simulink model "IEEEG1_unitStepResponse"  (R2022a)
settings: Solver=VariableStepAuto  StartTime=0.0  StopTime=t_sim  RelTol=1e-3
undefined symbols (not defined in the file or in its folder): K, K1, K3, K5, K7, T1, T2, T3, T4, T5, T6, T7
settings Model: Creator=jongoh  LastModifiedBy=jongoh

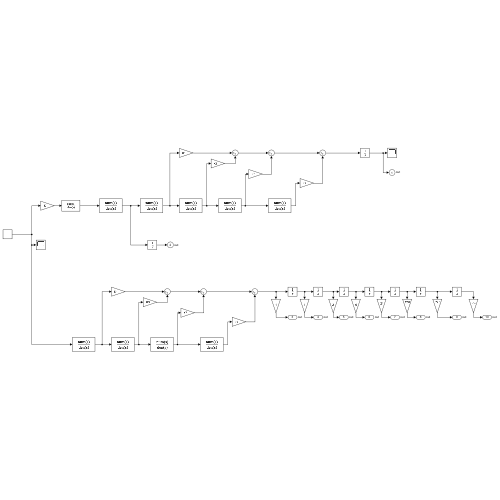
[thumbnail: Simulink's stored preview of the top-level diagram]
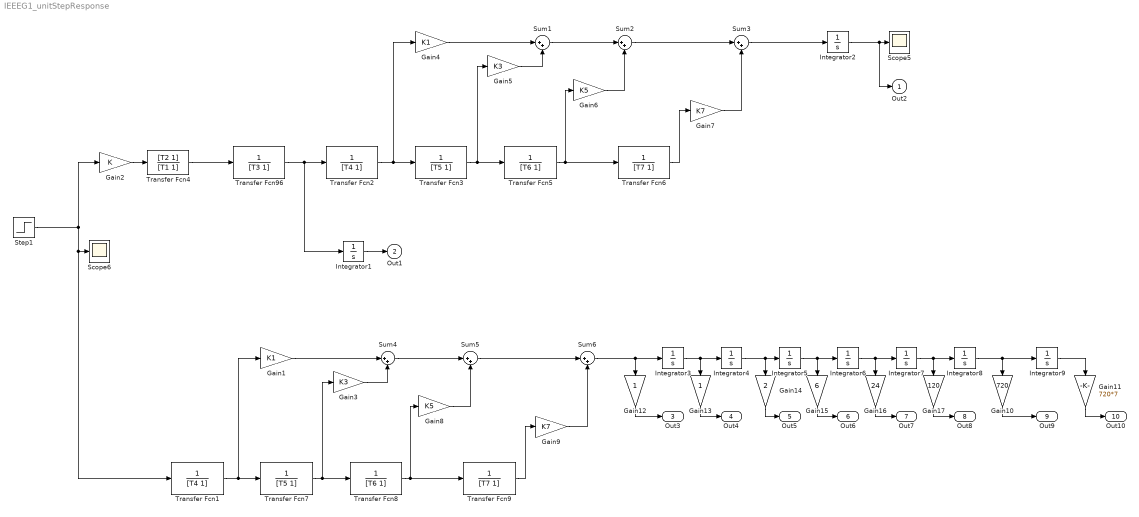
== system IEEEG1_unitStepResponse ==
  Gain1 : Gain  Gain=K1
  Gain10 : Gain  Gain=720
  Gain11 : Gain  Gain=720*7
  Gain12 : Gain
  Gain13 : Gain
  Gain14 : Gain  Gain=2
  Gain15 : Gain  Gain=6
  Gain16 : Gain  Gain=24
  Gain17 : Gain  Gain=120
  Gain2 : Gain  Gain=K
  Gain3 : Gain  Gain=K3
  Gain4 : Gain  Gain=K1
  Gain5 : Gain  Gain=K3
  Gain6 : Gain  Gain=K5
  Gain7 : Gain  Gain=K7
  Gain8 : Gain  Gain=K5
  Gain9 : Gain  Gain=K7
  Integrator{1..9} (9 alike) : Integrator
  Scope5 : Scope
  Scope6 : Scope
  Step1 : Step  Time=0  SampleTime=0
  Sum{1..6} (6 alike) : Sum  Inputs=|++
  Transfer Fcn1 : TransferFcn  Denominator=[T4 1]
  Transfer Fcn2 : TransferFcn  Denominator=[T4 1]
  Transfer Fcn3 : TransferFcn  Denominator=[T5 1]
  Transfer Fcn4 : TransferFcn  Numerator=[T2 1]  Denominator=[T1 1]
  Transfer Fcn5 : TransferFcn  Denominator=[T6 1]
  Transfer Fcn6 : TransferFcn  Denominator=[T7 1]
  Transfer Fcn7 : TransferFcn  Denominator=[T5 1]
  Transfer Fcn8 : TransferFcn  Denominator=[T6 1]
  Transfer Fcn9 : TransferFcn  Denominator=[T7 1]
  Transfer Fcn96 : TransferFcn  Denominator=[T3 1]
  Out2 : Outport  SignalName=out
  Out1 : Outport  Port=2  SignalName=out
  Out3 : Outport  Port=3  SignalName=out
  Out4 : Outport  Port=4  SignalName=out
  Out5 : Outport  Port=5  SignalName=out
  Out6 : Outport  Port=6  SignalName=out
  Out7 : Outport  Port=7  SignalName=out
  Out8 : Outport  Port=8  SignalName=out
  Out9 : Outport  Port=9  SignalName=out
  Out10 : Outport  Port=10  SignalName=out
  wires:
  Transfer Fcn2/1 -> Gain4/1, Transfer Fcn3/1
  Sum1/1 -> Sum2/1
  Transfer Fcn6/1 -> Gain7/1
  Gain6/1 -> Sum2/2
  Gain4/1 -> Sum1/1
  Gain2/1 -> Transfer Fcn4/1
  Sum3/1 -> Integrator2/1
  Gain7/1 -> Sum3/2
  Transfer Fcn96/1 -> Integrator1/1, Transfer Fcn2/1
  Step1/1 -> Transfer Fcn1/1, Scope6/1, Gain2/1
  Transfer Fcn4/1 -> Transfer Fcn96/1
  Transfer Fcn3/1 -> Gain5/1, Transfer Fcn5/1
  Transfer Fcn5/1 -> Gain6/1, Transfer Fcn6/1
  Gain5/1 -> Sum1/2
  Sum2/1 -> Sum3/1
  Integrator2/1 -> Out2/1, Scope5/1
  Integrator1/1 -> Out1/1
  Gain3/1 -> Sum4/2
  Sum5/1 -> Sum6/1
  Transfer Fcn1/1 -> Gain1/1, Transfer Fcn7/1
  Gain1/1 -> Sum4/1
  Transfer Fcn7/1 -> Gain3/1, Transfer Fcn8/1
  Gain9/1 -> Sum6/2
  Sum4/1 -> Sum5/1
  Gain8/1 -> Sum5/2
  Transfer Fcn9/1 -> Gain9/1
  Transfer Fcn8/1 -> Gain8/1, Transfer Fcn9/1
  Gain12/1 -> Out3/1
  Gain10/1 -> Out9/1
  Integrator9/1 -> Gain11/1
  Gain17/1 -> Out8/1
  Sum6/1 -> Gain12/1, Integrator3/1
  Gain15/1 -> Out6/1
  Integrator7/1 -> Gain17/1, Integrator8/1
  Gain16/1 -> Out7/1
  Gain13/1 -> Out4/1
  Integrator6/1 -> Gain16/1, Integrator7/1
  Gain14/1 -> Out5/1
  Integrator8/1 -> Gain10/1, Integrator9/1
  Integrator4/1 -> Gain14/1, Integrator5/1
  Integrator3/1 -> Gain13/1, Integrator4/1
  Integrator5/1 -> Gain15/1, Integrator6/1
  Gain11/1 -> Out10/1
